simulink model "First_Model"  (R2021b)
settings: Solver=ode4  StartTime=0.0  StopTime=0.2  FixedStep=10^-5  RelTol=1e-3
settings Model: Creator=amr_y  LastModifiedBy=amr_y

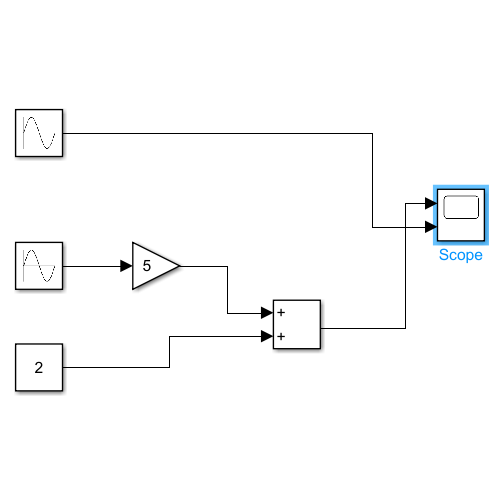
[thumbnail: Simulink's stored preview of the top-level diagram]
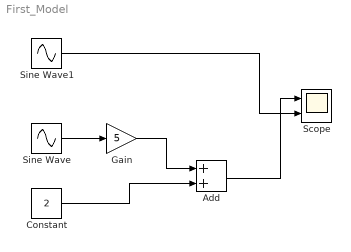
== system First_Model ==
  Add : Sum
  Constant : Constant  Value=2
  Gain : Gain  Gain=5
  Scope : Scope  NumInputPorts=2
  Sine Wave : Sin  Frequency=50  SampleTime=0
  Sine Wave1 : Sin  Amplitude=5  Bias=2  Frequency=50  Phase=-pi/2  SampleTime=0
  wires:
  Sine Wave/1 -> Gain/1
  Gain/1 -> Add/1
  Constant/1 -> Add/2
  Add/1 -> Scope/1
  Sine Wave1/1 -> Scope/2
